simulink subsystem "DC_Motor"  (R2022b)
settings: Solver=VariableStepAuto  StartTime=0.0  StopTime=10.0  RelTol=1e-3
model mask{Km=0, Kw=0, R=0, L=0, J_engine=0}
  mask prompts: Km "Motor torque constant"; Kw "Motor speed constant"; R "Armature resistance"; L "Armature inductance"; J_engine "Armature moment of inertia"
settings Model: Creator=Maxim Kozlov  LastModifiedBy=Maxim Kozlov
settings OptimizationCC: ReuseModelBlockBuffer=on

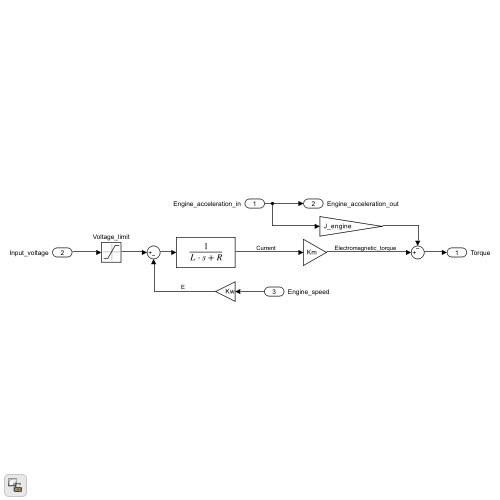
[thumbnail: Simulink's stored preview of the top-level diagram]
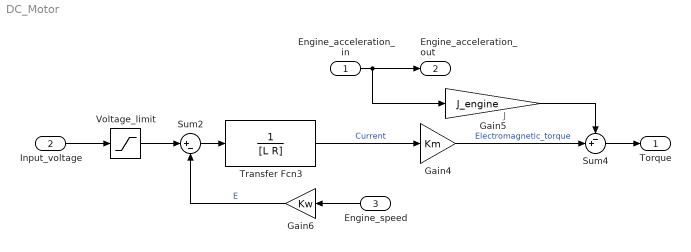
== system DC_Motor ==
  note: J
  Engine_acceleration_in : Inport
  Input_voltage : Inport  Port=2
  Engine_speed : Inport  Port=3
  Gain4 : Gain  Gain=Km
  Gain5 : Gain  Gain=J_engine
  Gain6 : Gain  Gain=Kw
  Sum2 : Sum  Inputs=|+-
  Sum4 : Sum  Inputs=-+|
  Transfer Fcn3 : TransferFcn  Denominator=[L R]
  Voltage_limit : Saturate  UpperLimit=10.8  LowerLimit=-10.8
  Torque : Outport
  Engine_acceleration_out : Outport  Port=2
  wires:
  Gain5/1 -> Sum4/1
  Gain4/1 -> Sum4/2  "Electromagnetic_torque"
  Engine_acceleration_in/1 -> Gain5/1, Engine_acceleration_out/1
  Sum2/1 -> Transfer Fcn3/1
  Gain6/1 -> Sum2/2  "E"
  Transfer Fcn3/1 -> Gain4/1  "Сurrent"
  Voltage_limit/1 -> Sum2/1
  Engine_speed/1 -> Gain6/1
  Sum4/1 -> Torque/1
  Input_voltage/1 -> Voltage_limit/1
